simulink subsystem "Motor"  (R2024b)
settings: Solver=VariableStepAuto  StartTime=0.0  StopTime=10.0  RelTol=1e-3
values from neighbouring files (symbols this model uses):
  K_b = 0.02    [D1script.m]    (also in disp.mat = 0.0301; onlabscript.m = 0.0301)
  K_t = 0.02    [D1script.m]    (also in disp.mat = 0.03; onlabscript.m = 0.03)
  La = 1.5e-3    (= 0.0015)    [D1script.m]    (also in disp.mat = 0.94; onlabscript.m = 0.94)
  Ra = 1.2    [D1script.m]    (also in disp.mat = 1; onlabscript.m = 1)
settings Model: Creator=Asus  LastModifiedBy=Asus

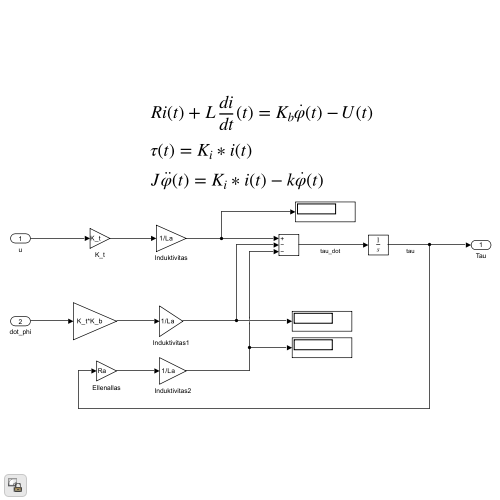
[thumbnail: Simulink's stored preview of the top-level diagram]
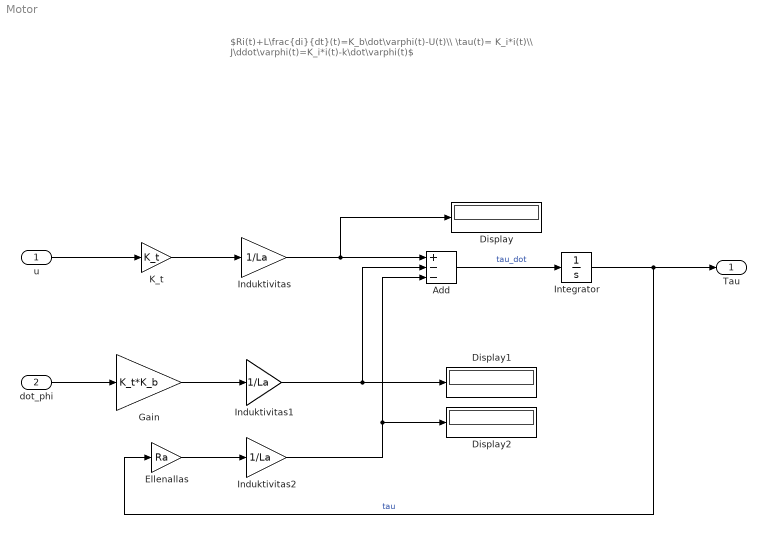
== system Motor ==
  note: $Ri(t)+L\frac{di}{dt}(t)=K_b\dot\varphi(t)-U(t)\\ \tau(t)= K_i*i(t)\\ J\ddot\varphi(t)=K_i*i(t)-k\dot\varphi(t)$
  u : Inport
  dot_phi : Inport  Port=2
  Add : Sum  Inputs=+--
  Display : Display
  Display1 : Display
  Display2 : Display
  Ellenallas : Gain  Gain=Ra
  Gain : Gain  Gain=K_t*K_b
  Induktivitas : Gain  Gain=1/La
  Induktivitas1 : Gain  Gain=1/La
  Induktivitas2 : Gain  Gain=1/La
  Integrator : Integrator
  K_t : Gain  Gain=K_t
  Tau : Outport
  wires:
  u/1 -> K_t/1
  K_t/1 -> Induktivitas/1
  dot_phi/1 -> Gain/1
  Gain/1 -> Induktivitas1/1
  Induktivitas1/1 -> Add/2, Display1/1
  Induktivitas/1 -> Add/1, Display/1
  Induktivitas2/1 -> Add/3, Display2/1
  Add/1 -> Integrator/1  "tau_dot"
  Integrator/1 -> Tau/1, Ellenallas/1  "tau"
  Ellenallas/1 -> Induktivitas2/1
